simulink model "sampleModel112"  (Simulink 9.1)
settings: Solver=VariableStepAuto  StartTime=0.0  StopTime=10.0  RelTol=1e-3
undefined symbols (not defined in the file): DiscIntNeverNeededParam, Newton, Raphson
libraries: simulink x44
(part 1 of 2)
settings Model: SuppressorTable="22 serialization::archive 11 0 6 0 0 1 8 0 0 0 0 6 0 0 1 0 22 sampleModel112/cfblk81 0 6 0 0 2 8 0 0 0 0 6 41 Simulink:DataType:WarningOverFlowDetected 0 0 0 6 0  0  0 0 0 0 8 20160608 0 0 0 15 23 17 0 1 40 SimulinkFixedPoint:util:Overflowoccurred 0 0 0  0  8 20160608 0 15 23 17 0 1"  Creator=DELL  LastModifiedBy=DELL
settings DataIOCC: SaveFormat=Dataset
settings OptimizationCC: LifeSpan=auto
settings DebuggingCC: UnderspecifiedInitializationDetection=Simplified  MergeDetectMultiDrivingBlocksExec=error  SFUnexpectedBacktrackingDiag=error  SFNoUnconditionalDefaultTransitionDiag=error  SFExecutionAtInitializationDiag=warning
settings HardwareCC: ProdBitPerPointer=64  ProdBitPerSizeT=64  ProdBitPerPtrDiffT=64  ProdLargestAtomicFloat=Float  ProdIntDivRoundTo=Zero  ProdEndianess=LittleEndian  ProdWordSize=64  ProdHWDeviceType=Intel->x86-64 (Windows64)
settings ModelReferenceCC: PropagateSignalLabelsOutOfModel=on
settings CodeAppCC: StateflowObjectComments=off
settings GRTTargetCC: TargetLangStandard=C99 (ISO)  CombineOutputUpdateFcns=on  GRTInterface=off
settings ConfigComp: CovMetricSettings=dwe  CovHtmlReporting=off  CovSaveCumulativeToWorkspaceVar=off  CovSaveSingleToWorkspaceVar=off  CovExternalEMLEnable=on

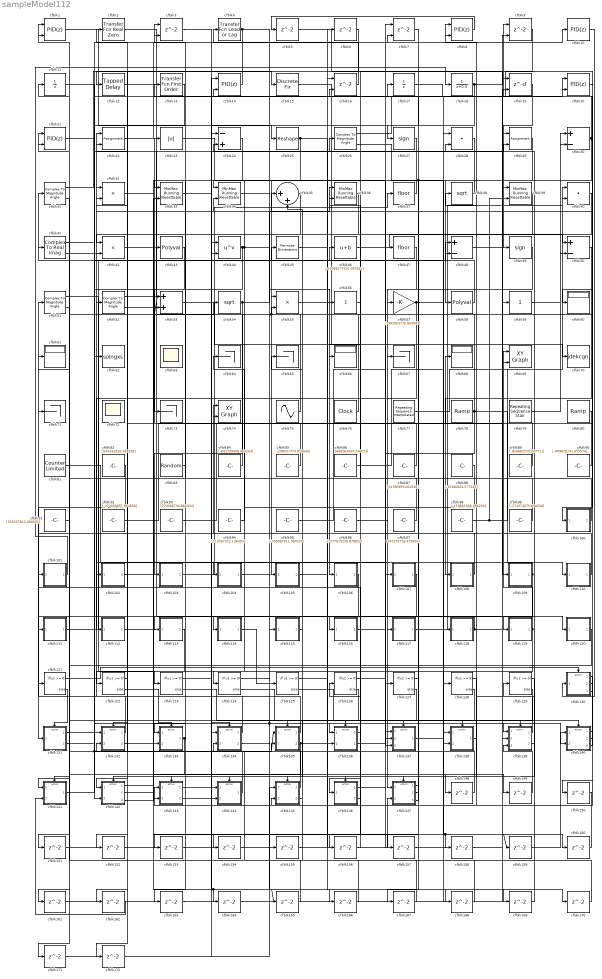
== system sampleModel112 ==
  cfblk{1,8,14,20..21} (5 alike) : simulink/Continuous/PID Controller (2DOF)  Controller=PID  TimeDomain=Discrete-time  SampleTime=1  IntegratorMethod=Forward Euler  FilterMethod=Forward Euler  Form=Parallel  UseFilter=on  ControllerParametersSource=internal  P=1  I=1  D=0  N=100  b=1  c=1  InitialConditionSource=internal  InitialConditionForIntegrator=0  InitialConditionForFilter=0  ExternalReset=none  LimitOutput=off  UpperSaturationLimit=inf  LowerSaturationLimit=-inf  LinearizeAsGain=off  AntiWindupMode=none  Kb=1  TrackingMode=off  Kt=1  PParamMin=[]  PParamMax=[]  IParamMin=[]  IParamMax=[]  DParamMin=[]  DParamMax=[]  NParamMin=[]  NParamMax=[]  bParamMin=[]  bParamMax=[]  cParamMin=[]  cParamMax=[]  KbParamMin=[]  KbParamMax=[]  KtParamMin=[]  KtParamMax=[]  POutMin=[]  POutMax=[]  IOutMin=[]  IOutMax=[]  DOutMin=[]  DOutMax=[]  NOutMin=[]  NOutMax=[]  bOutMin=[]  bOutMax=[]  cOutMin=[]  cOutMax=[]  KbOutMin=[]  KbOutMax=[]  KtOutMin=[]  KtOutMax=[]  IntegratorOutMin=[]  IntegratorOutMax=[]  FilterOutMin=[]  FilterOutMax=[]  SumOutMin=[]  SumOutMax=[]  Sum1OutMin=[]  Sum1OutMax=[]  Sum2OutMin=[]  Sum2OutMax=[]  Sum3OutMin=[]  Sum3OutMax=[]  SumI1OutMin=[]  SumI1OutMax=[]  SumI2OutMin=[]  SumI2OutMax=[]  SumI3OutMin=[]  SumI3OutMax=[]  SumDOutMin=[]  SumDOutMax=[]  SaturationOutMin=[]  SaturationOutMax=[]  IntegratorContinuousStateAttributes=''  IntegratorStateMustResolveToSignalObject=off  IntegratorRTWStateStorageClass=Auto  FilterContinuousStateAttributes=''  FilterStateMustResolveToSignalObject=off  FilterRTWStateStorageClass=Auto  DifferentiatorICPrevScaledInput=0  DifferentiatorOutMin=[]  DifferentiatorOutMax=[]  FilterDiffOutCoefMin=[]  FilterDiffOutCoefMax=[]  SumDenOutMin=[]  SumDenOutMax=[]  SumNumOutMin=[]  SumNumOutMax=[]  ReciprocalOutMin=[]  ReciprocalOutMax=[]  DivideOutMin=[]  DivideOutMax=[]  TunerSelectOption=Transfer Function Based (PID Tuner App)
  cfblk10 : simulink/Continuous/PID Controller  Controller=PID  TimeDomain=Discrete-time  SampleTime=1  IntegratorMethod=Forward Euler  FilterMethod=Forward Euler  Form=Parallel  UseFilter=on  ControllerParametersSource=internal  P=1  I=1  D=0  N=100  InitialConditionSource=internal  InitialConditionForIntegrator=0  InitialConditionForFilter=0  ExternalReset=none  LimitOutput=off  UpperSaturationLimit=inf  LowerSaturationLimit=-inf  LinearizeAsGain=off  AntiWindupMode=none  Kb=1  TrackingMode=off  Kt=1  PParamMin=[]  PParamMax=[]  IParamMin=[]  IParamMax=[]  DParamMin=[]  DParamMax=[]  NParamMin=[]  NParamMax=[]  KbParamMin=[]  KbParamMax=[]  KtParamMin=[]  KtParamMax=[]  POutMin=[]  POutMax=[]  IOutMin=[]  IOutMax=[]  DOutMin=[]  DOutMax=[]  NOutMin=[]  NOutMax=[]  KbOutMin=[]  KbOutMax=[]  KtOutMin=[]  KtOutMax=[]  IntegratorOutMin=[]  IntegratorOutMax=[]  FilterOutMin=[]  FilterOutMax=[]  SumOutMin=[]  SumOutMax=[]  SumI1OutMin=[]  SumI1OutMax=[]  SumI2OutMin=[]  SumI2OutMax=[]  SumI3OutMin=[]  SumI3OutMax=[]  SumDOutMin=[]  SumDOutMax=[]  SaturationOutMin=[]  SaturationOutMax=[]  IntegratorContinuousStateAttributes=''  IntegratorStateMustResolveToSignalObject=off  IntegratorRTWStateStorageClass=Auto  FilterContinuousStateAttributes=''  FilterStateMustResolveToSignalObject=off  FilterRTWStateStorageClass=Auto  DifferentiatorICPrevScaledInput=0  DifferentiatorOutMin=[]  DifferentiatorOutMax=[]  FilterDiffOutCoefMin=[]  FilterDiffOutCoefMax=[]  SumDenOutMin=[]  SumDenOutMax=[]  SumNumOutMin=[]  SumNumOutMax=[]  ReciprocalOutMin=[]  ReciprocalOutMax=[]  DivideOutMin=[]  DivideOutMax=[]  TunerSelectOption=Transfer Function Based (PID Tuner App)
  cfblk100 : Subsystem
  cfblk101 : Subsystem
  cfblk102 : Subsystem
  cfblk103 : Subsystem
  cfblk104 : Subsystem
  cfblk105 : Subsystem
  cfblk106 : Subsystem
  cfblk107 : Subsystem
  cfblk108 : Subsystem
  cfblk109 : Subsystem
  cfblk11 : UnitDelay
  cfblk110 : Subsystem
  cfblk111 : Subsystem
  cfblk112 : Subsystem
  cfblk113 : Subsystem
  cfblk114 : Subsystem
  cfblk115 : Subsystem
  cfblk116 : Subsystem
  cfblk117 : Subsystem
  cfblk118 : Subsystem
  cfblk119 : Subsystem
  cfblk12 : simulink/Discrete/Tapped Delay  vinit=0.0  samptime=-1  NumDelays=1  DelayOrder=Oldest  includeCurrent=off
  cfblk120 : Subsystem
  cfblk{121..129} (9 alike) : If  IfExpression=u1 >= 0  SampleTime=1
  cfblk13 : simulink/Discrete/Transfer Fcn First Order  PoleZ=0.95  ICPrevOutput=0.0  DoSatur=off
      settings: SourceProductName=Simulink
  cfblk130 : Subsystem  TreatAsAtomicUnit=on
  cfblk131 : Subsystem  TreatAsAtomicUnit=on
  cfblk132 : Subsystem  TreatAsAtomicUnit=on
  cfblk133 : Subsystem  TreatAsAtomicUnit=on
  cfblk134 : Subsystem  TreatAsAtomicUnit=on
  cfblk135 : Subsystem  TreatAsAtomicUnit=on
  cfblk136 : Subsystem  TreatAsAtomicUnit=on
  cfblk137 : Subsystem  TreatAsAtomicUnit=on
  cfblk138 : Subsystem  TreatAsAtomicUnit=on
  cfblk139 : Subsystem  TreatAsAtomicUnit=on
  cfblk140 : Subsystem  TreatAsAtomicUnit=on
  cfblk141 : Subsystem  TreatAsAtomicUnit=on
  cfblk142 : Subsystem  TreatAsAtomicUnit=on
  cfblk143 : Subsystem  TreatAsAtomicUnit=on
  cfblk144 : Subsystem  TreatAsAtomicUnit=on
  cfblk145 : Subsystem  TreatAsAtomicUnit=on
  cfblk146 : Subsystem  TreatAsAtomicUnit=on
  cfblk147 : Subsystem  TreatAsAtomicUnit=on
  cfblk{5..6,148..172} (27 alike) : Delay  SampleTime=1
  cfblk15 : DiscreteFir  SampleTime=1
  cfblk{3,7,9,16} (4 alike) : Delay  ShowEnablePort=on  SampleTime=1
      settings: InputPortMap=u0,e6
  cfblk17 : UnitDelay
  cfblk18 : DiscreteTransferFcn  SampleTime=1
  cfblk19 : Delay  DelayLengthSource=Input port  SampleTime=1
      settings: InputPortMap=u0,p1
  cfblk2 : simulink/Discrete/Transfer Fcn Real Zero  ZeroZ=0.75  ICPrevInput=0.0  DoSatur=off
      settings: SourceProductName=Simulink  SourceProductBaseCode=SL
  cfblk22 : Assignment  DiagnosticForDimensions=Warning  IndexOptions=Index vector (dialog)  Indices=1  OutputSizes=1
  cfblk23 : Abs
  cfblk24 : Sum  Inputs=-+
  cfblk25 : Reshape
  cfblk{26,31,51..52} (4 alike) : ComplexToMagnitudeAngle
  cfblk27 : Signum
  cfblk28 : DotProduct  InputSameDT=on  OutDataTypeStr=Inherit: Inherit via internal rule
  cfblk29 : Assignment  DiagnosticForDimensions=Warning  IndexOptions=Index vector (dialog)  Indices=1  OutputSizes=1
  cfblk30 : Sum  Inputs=+-
  cfblk32 : Product
  cfblk{33..34,36,39} (4 alike) : simulink/Math Operations/MinMax Running Resettable  Function=min  vinit=0.0
  cfblk35 : Sum  Inputs=|++
  cfblk37 : Rounding
  cfblk38 : Sqrt  SaturateOnIntegerOverflow=on
  cfblk4 : simulink/Discrete/Transfer Fcn Lead or Lag  PoleZ=0.95  ZeroZ=0.75  ICPrevOutput=0.0  ICPrevInput=0.0  DoSatur=off
      settings: SourceProductName=Simulink  SourceProductBaseCode=SL
  cfblk40 : DotProduct  InputSameDT=on  OutDataTypeStr=Inherit: Inherit via internal rule
  cfblk41 : ComplexToRealImag
  cfblk42 : Product  Inputs=**
  cfblk43 : Polyval  Coefs=[ +2.081618890e-019, -1.441693666e-014, +4.719686976e-010, -8.536869453e-006, +1.621573104e-001, -8.087801117e+001 ]
  cfblk44 : Math  Operator=pow  SaturateOnIntegerOverflow=on
  cfblk45 : PermuteDimensions
  cfblk46 : Bias  Bias=[989277410.097821]
  cfblk47 : Rounding
  cfblk48 : Sum  Inputs=+-
  cfblk49 : Signum
  cfblk50 : Sum  Inputs=+-
  cfblk53 : Sum
  cfblk54 : Sqrt  SaturateOnIntegerOverflow=on
  cfblk55 : Product  Inputs=**
  cfblk56 : Sum  Inputs=+
  cfblk57 : Gain  Gain=[-992003770.603943]
  cfblk58 : Polyval  Coefs=[ +2.081618890e-019, -1.441693666e-014, +4.719686976e-010, -8.536869453e-006, +1.621573104e-001, -8.087801117e+001 ]
  cfblk59 : simulink/Math Operations/Slider Gain  gain=1  low=0  high=2
  cfblk{60..61,66,68} (4 alike) : Display
  cfblk62 : ToWorkspace  VariableName=solngxs  SaveFormat=Timeseries  SampleTime=-1
  cfblk63 : Scope
      settings: Floating=on
  cfblk{64..65,67,71,73} (5 alike) : Terminator
  cfblk69 : simulink/Sinks/XY Graph  xmin=-1  xmax=1  ymin=-1  ymax=1  st=-1
  cfblk70 : ToWorkspace  VariableName=jdekcgn  SaveFormat=Timeseries  SampleTime=-1
  cfblk72 : Scope
      settings: Floating=on
  cfblk74 : simulink/Sinks/XY Graph  xmin=-1  xmax=1  ymin=-1  ymax=1  st=-1
  cfblk75 : Sin  Amplitude=[-145605885.382859]  Bias=[-797728255.211016]  SampleTime=0
  cfblk76 : DigitalClock
  cfblk77 : simulink/Sources/Repeating Sequence Interpolated  OutValues=[-370249542.565422, -774787693.113988, 675281554.388704, -493341960.193509, 181293686.473387]  TimeValues=[0 0.1 0.5 0.6 1].'  LookUpMeth=Use Input Above  tsamp=0.01  OutMin=[]  OutMax=[]  OutDataTypeStr=double  OutputDataTypeScalingMode=double  OutDataType=fixdt(0,8)  OutScaling=2^-10
  cfblk78 : simulink/Sources/Ramp  slope=[2818.028998]  start=[30.439824]  InitialOutput=[315717.012690]
  cfblk79 : simulink/Sources/Repeating Sequence Stair  OutValues=[132599061.622461, -803275858.841919]  tsamp=-1  OutMin=[]  OutMax=[]  OutDataTypeStr=double  OutputDataTypeScalingMode=double  OutDataType=fixdt(0,8)  ConRadixGroup=Best Precision: Vector-wise  OutScaling=2^-12
  cfblk80 : simulink/Sources/Ramp  slope=[-5793.235328]  start=[14.690566]  InitialOutput=[133772.427561]
  cfblk81 : simulink/Sources/Counter Limited  uplimit=[276.000000]  tsamp=-1
  cfblk82 : Constant  Value=[639181520.339358]  SampleTime=1
  cfblk83 : UniformRandomNumber  Minimum=[-8236368095.741834]  Maximum=[8276593604.768766]  Seed=[22727342.000000]  SampleTime=0.1
  cfblk84 : Constant  Value=[-641739458.403204]  SampleTime=1
  cfblk85 : Constant  Value=[298537775.810636]  SampleTime=1
  cfblk86 : Constant  Value=[448583934.246073]  SampleTime=1
  cfblk87 : Constant  Value=[54786959.062546]  SampleTime=1
  cfblk88 : Constant  Value=[-19180664.577623]  SampleTime=1
  cfblk89 : Constant  Value=[-826682570.047711]  SampleTime=1
  cfblk90 : Constant  Value=[-989820241.655576]  SampleTime=1
  cfblk91 : Constant  Value=[555557812.090935]  SampleTime=1
  cfblk92 : Constant  Value=[-274050697.954858]  SampleTime=1
  cfblk93 : Constant  Value=[270266734.884034]  SampleTime=1
  cfblk94 : Constant  Value=[113067322.136453]  SampleTime=1
  cfblk95 : Constant  Value=[-750967911.584239]  SampleTime=1
  cfblk96 : Constant  Value=[-277615226.876852]  SampleTime=1
  cfblk97 : Constant  Value=[497279716.475859]  SampleTime=1
  cfblk98 : Constant  Value=[-119851956.386200]  SampleTime=1
  cfblk99 : Constant  Value=[-174374075.858508]  SampleTime=1
  wires:
  cfblk27/1 -> cfblk105/1(cfblk1)
  cfblk12/1 -> cfblk120/1(cfblk1)
  cfblk114/1(cfblk2) -> cfblk125/1
  cfblk132/1(cfblk2) -> cfblk22/1
  cfblk77/1 -> cfblk40/1
  cfblk108/1(cfblk2) -> cfblk51/1
  cfblk31/1 -> cfblk15/1
  cfblk37/1 -> cfblk34/1
  cfblk113/1(cfblk2) -> cfblk122/1
  cfblk96/1 -> cfblk147/1(cfblk1)
  cfblk54/1 -> cfblk103/1(cfblk1), cfblk36/2
  cfblk55/1 -> cfblk106/1(cfblk1)
  cfblk47/1 -> cfblk117/1(cfblk1)
  cfblk19/1 -> cfblk49/1
  cfblk101/1(cfblk2) -> cfblk18/1
  cfblk143/1(cfblk2) -> cfblk17/1
  cfblk102/1(cfblk2) -> cfblk164/1, cfblk165/1
  cfblk16/1 -> cfblk4/1
  cfblk81/1 -> cfblk127/1
  cfblk117/1(cfblk2) -> cfblk40/2
  cfblk53/1 -> cfblk67/1
  cfblk38/1 -> cfblk58/1
  cfblk92/1 -> cfblk68/1
  cfblk140/1(cfblk2) -> cfblk143/1(cfblk1)
  cfblk30/1 -> cfblk143/2(cfblk14), cfblk16/2
  cfblk103/1(cfblk2) -> cfblk37/1
  cfblk17/1 -> cfblk100/1(cfblk1)
  cfblk1/1 -> cfblk115/1(cfblk1)
  cfblk15/1 -> cfblk70/1
  cfblk9/1 -> cfblk66/1
  cfblk35/1 -> cfblk42/1
  cfblk111/1(cfblk2) -> cfblk48/1
  cfblk26/1 -> cfblk9/1
  cfblk131/1(cfblk2) -> cfblk132/1(cfblk1)
  cfblk2/1 -> cfblk25/1
  cfblk146/1(cfblk2) -> cfblk137/1(cfblk1)
  cfblk82/1 -> cfblk131/1(cfblk1)
  cfblk134/1(cfblk2) -> cfblk71/1
  cfblk7/1 -> cfblk27/1
  cfblk105/1(cfblk2) -> cfblk48/2
  cfblk86/1 -> cfblk28/1
  cfblk97/1 -> cfblk46/1
  cfblk20/1 -> cfblk60/1
  cfblk58/1 -> cfblk31/1
  cfblk109/1(cfblk2) -> cfblk121/1, cfblk102/1(cfblk1)
  cfblk107/1(cfblk2) -> cfblk111/1(cfblk1)
  cfblk110/1(cfblk2) -> cfblk74/1
  cfblk23/1 -> cfblk107/1(cfblk1)
  cfblk89/1 -> cfblk36/1
  cfblk79/1 -> cfblk30/1
  cfblk85/1 -> cfblk23/1
  cfblk14/1 -> cfblk12/1
  cfblk4/1 -> cfblk56/1, cfblk152/1
  cfblk39/1 -> cfblk146/1(cfblk1)
  cfblk138/1(cfblk2) -> cfblk38/1
  cfblk84/1 -> cfblk32/1
  cfblk8/1 -> cfblk5/1
  cfblk51/1 -> cfblk123/1
  cfblk3/1 -> cfblk119/1(cfblk1)
  cfblk25/1 -> cfblk144/2(cfblk9), cfblk140/2(cfblk11)
  cfblk146/2(cfblk7) -> cfblk101/1(cfblk1)
  cfblk99/1 -> cfblk3/1
  cfblk51/2 -> cfblk11/1
  cfblk43/1 -> cfblk73/1
  cfblk143/2(cfblk15) -> cfblk14/1
  cfblk147/3(cfblk14) -> cfblk13/1
  cfblk10/1 -> cfblk130/1(cfblk1)
  cfblk46/1 -> cfblk50/1
  cfblk48/1 -> cfblk59/1
  cfblk40/1 -> cfblk55/1
  cfblk50/1 -> cfblk108/1(cfblk1)
  cfblk11/1 -> cfblk62/1
  cfblk13/1 -> cfblk42/2
  cfblk94/1 -> cfblk64/1
  cfblk29/1 -> cfblk104/1(cfblk1), cfblk167/1
  cfblk88/1 -> cfblk124/1
  cfblk93/1 -> cfblk69/1
  cfblk28/1 -> cfblk113/1(cfblk1)
  cfblk131/2(cfblk10) -> cfblk3/2
  cfblk119/1(cfblk2) -> cfblk69/2, cfblk133/2(cfblk7)
  cfblk87/1 -> cfblk22/2
  cfblk59/1 -> cfblk30/2
  cfblk41/1 -> cfblk136/1(cfblk1)
  cfblk115/1(cfblk2) -> cfblk35/2
  cfblk6/1 -> cfblk142/1(cfblk1)
  cfblk41/2 -> cfblk19/1
  cfblk118/1(cfblk2) -> cfblk39/1, cfblk116/1(cfblk1)
  cfblk52/1 -> cfblk26/1
  cfblk5/1 -> cfblk109/1(cfblk1)
  cfblk112/1(cfblk2) -> cfblk158/1, cfblk159/1
  cfblk136/1(cfblk2) -> cfblk132/2(cfblk14)
  cfblk44/1 -> cfblk114/1(cfblk1), cfblk139/1(cfblk1), cfblk142/2(cfblk14)
  cfblk78/1 -> cfblk110/1(cfblk1), cfblk137/3(cfblk13), cfblk53/2
  cfblk90/1 -> cfblk28/2
  cfblk76/1 -> cfblk1/1
  cfblk144/1(cfblk2) -> cfblk52/1
  cfblk98/1 -> cfblk50/2, cfblk39/2
  cfblk22/1 -> cfblk7/2
  cfblk145/1(cfblk2) -> cfblk41/1
  cfblk26/2 -> cfblk118/1(cfblk1)
  cfblk21/1 -> cfblk29/2
  cfblk116/1(cfblk2) -> cfblk10/1
  cfblk136/2(cfblk15) -> cfblk20/1
  cfblk130/2(cfblk6) -> cfblk32/2
  cfblk57/1 -> cfblk112/1(cfblk1), cfblk160/1
  cfblk95/1 -> cfblk47/1
  cfblk24/1 -> cfblk33/1
  cfblk142/1(cfblk2) -> cfblk33/2
  cfblk140/2(cfblk12) -> cfblk34/2
  cfblk75/1 -> cfblk2/1
  cfblk141/1(cfblk2) -> cfblk43/1, cfblk135/1(cfblk1)
  cfblk100/1(cfblk2) -> cfblk1/2
  cfblk145/2(cfblk15) -> cfblk65/1
  cfblk140/3(cfblk13) -> cfblk14/2
  cfblk137/1(cfblk2) -> cfblk20/2
  cfblk32/1 -> cfblk136/2(cfblk14)
  cfblk80/1 -> cfblk74/2
  cfblk142/3(cfblk16) -> cfblk45/1
  cfblk139/1(cfblk2) -> cfblk8/1
  cfblk49/1 -> cfblk57/1
  cfblk91/1 -> cfblk61/1
  cfblk52/2 -> cfblk54/1
  cfblk18/1 -> cfblk9/2, cfblk44/2
  cfblk139/2(cfblk17) -> cfblk24/2
  cfblk130/3(cfblk7) -> cfblk53/1, cfblk55/2
  cfblk135/1(cfblk2) -> cfblk21/1
  cfblk135/2(cfblk10) -> cfblk6/1, cfblk171/1
  cfblk31/2 -> cfblk141/1(cfblk1)
  cfblk104/1(cfblk2) -> cfblk137/2(cfblk12), cfblk149/1
  cfblk83/1 -> cfblk133/1(cfblk1)
  cfblk133/1(cfblk2) -> cfblk162/1, cfblk163/1
  cfblk121/1 -> cfblk130/Action
  cfblk121/2 -> cfblk131/Action
  cfblk122/1 -> cfblk132/Action
  cfblk122/2 -> cfblk133/Action
  cfblk123/1 -> cfblk134/Action
  cfblk123/2 -> cfblk135/Action
  cfblk124/1 -> cfblk136/Action
  cfblk124/2 -> cfblk137/Action
  cfblk125/1 -> cfblk138/Action
  cfblk125/2 -> cfblk139/Action
  cfblk126/1 -> cfblk140/Action
  cfblk126/2 -> cfblk141/Action
  cfblk127/1 -> cfblk142/Action
  cfblk127/2 -> cfblk143/Action
  cfblk128/1 -> cfblk144/Action
  cfblk128/2 -> cfblk145/Action
  cfblk129/1 -> cfblk146/Action
  cfblk129/2 -> cfblk147/Action
  cfblk42/1 -> cfblk148/1
  cfblk148/1 -> cfblk35/1
  cfblk149/1 -> cfblk139/3(cfblk16)
  cfblk130/1(cfblk2) -> cfblk150/1
  cfblk150/1 -> cfblk145/2(cfblk14)
  cfblk120/1(cfblk2) -> cfblk151/1
  cfblk151/1 -> cfblk128/1
  cfblk152/1 -> cfblk147/2(cfblk12)
  cfblk147/1(cfblk2) -> cfblk153/1
  cfblk153/1 -> cfblk138/2(cfblk7)
  cfblk147/2(cfblk13) -> cfblk154/1
  cfblk154/1 -> cfblk7/1
  cfblk34/1 -> cfblk155/1
  cfblk155/1 -> cfblk16/1
  cfblk56/1 -> cfblk156/1
  cfblk156/1 -> cfblk126/1
  cfblk132/2(cfblk15) -> cfblk157/1
  cfblk157/1 -> cfblk29/1
  cfblk158/1 -> cfblk19/2
  cfblk159/1 -> cfblk140/1(cfblk1)
  cfblk160/1 -> cfblk8/2
  cfblk106/1(cfblk2) -> cfblk161/1
  cfblk161/1 -> cfblk144/1(cfblk1)
  cfblk162/1 -> cfblk141/2(cfblk8)
  cfblk163/1 -> cfblk139/2(cfblk15)
  cfblk164/1 -> cfblk138/1(cfblk1)
  cfblk165/1 -> cfblk21/2
  cfblk33/1 -> cfblk166/1
  cfblk166/1 -> cfblk24/1
  cfblk167/1 -> cfblk135/2(cfblk9)
  cfblk142/2(cfblk15) -> cfblk168/1
  cfblk168/1 -> cfblk134/2(cfblk8)
  cfblk134/2(cfblk9) -> cfblk169/1
  cfblk169/1 -> cfblk129/1
  cfblk45/1 -> cfblk170/1
  cfblk170/1 -> cfblk134/1(cfblk1)
  cfblk171/1 -> cfblk44/1
  cfblk36/1 -> cfblk172/1
  cfblk172/1 -> cfblk145/1(cfblk1)

== system sampleModel112/cfblk100 ==
  cfblk1 : Inport
  cfblk2 : Outport
  wires:
  cfblk1/1 -> cfblk2/1

== system sampleModel112/cfblk101 ==
  cfblk1 : Inport
  cfblk2 : Outport
  wires:
  cfblk1/1 -> cfblk2/1

== system sampleModel112/cfblk102 ==
  cfblk1 : Inport
  cfblk2 : Outport
  wires:
  cfblk1/1 -> cfblk2/1

== system sampleModel112/cfblk103 ==
  cfblk1 : Inport
  cfblk2 : Outport
  wires:
  cfblk1/1 -> cfblk2/1

== system sampleModel112/cfblk104 ==
  cfblk1 : Inport
  cfblk2 : Outport
  wires:
  cfblk1/1 -> cfblk2/1

== system sampleModel112/cfblk105 ==
  cfblk1 : Inport
  cfblk2 : Outport
  wires:
  cfblk1/1 -> cfblk2/1

== system sampleModel112/cfblk106 ==
  cfblk1 : Inport
  cfblk2 : Outport
  wires:
  cfblk1/1 -> cfblk2/1

== system sampleModel112/cfblk107 ==
  cfblk1 : Inport
  cfblk2 : Outport
  wires:
  cfblk1/1 -> cfblk2/1

== system sampleModel112/cfblk108 ==
  cfblk1 : Inport
  cfblk2 : Outport
  wires:
  cfblk1/1 -> cfblk2/1

== system sampleModel112/cfblk109 ==
  cfblk1 : Inport
  cfblk2 : Outport
  wires:
  cfblk1/1 -> cfblk2/1

== system sampleModel112/cfblk110 ==
  cfblk1 : Inport
  cfblk2 : Outport
  wires:
  cfblk1/1 -> cfblk2/1

== system sampleModel112/cfblk111 ==
  cfblk1 : Inport
  cfblk2 : Outport
  wires:
  cfblk1/1 -> cfblk2/1

== system sampleModel112/cfblk112 ==
  cfblk1 : Inport
  cfblk2 : Outport
  wires:
  cfblk1/1 -> cfblk2/1

== system sampleModel112/cfblk113 ==
  cfblk1 : Inport
  cfblk2 : Outport
  wires:
  cfblk1/1 -> cfblk2/1

== system sampleModel112/cfblk114 ==
  cfblk1 : Inport
  cfblk2 : Outport
  wires:
  cfblk1/1 -> cfblk2/1

== system sampleModel112/cfblk115 ==
  cfblk1 : Inport
  cfblk2 : Outport
  wires:
  cfblk1/1 -> cfblk2/1

== system sampleModel112/cfblk116 ==
  cfblk1 : Inport
  cfblk2 : Outport
  wires:
  cfblk1/1 -> cfblk2/1

== system sampleModel112/cfblk117 ==
  cfblk1 : Inport
  cfblk2 : Outport
  wires:
  cfblk1/1 -> cfblk2/1

== system sampleModel112/cfblk118 ==
  cfblk1 : Inport
  cfblk2 : Outport
  wires:
  cfblk1/1 -> cfblk2/1

== system sampleModel112/cfblk119 ==
  cfblk1 : Inport
  cfblk2 : Outport
  wires:
  cfblk1/1 -> cfblk2/1

== system sampleModel112/cfblk120 ==
  cfblk1 : Inport
  cfblk2 : Outport
  wires:
  cfblk1/1 -> cfblk2/1

== system sampleModel112/cfblk130 ==
  cfblk1 : Inport
  Action Port : ActionPort  ActionType=then
  cfblk3 : ComplexToRealImag
  cfblk4 : Sqrt  Operator=rSqrt  AlgorithmType=Newton-Raphson  SaturateOnIntegerOverflow=on
  cfblk5 : Subsystem
  cfblk2 : Outport
  cfblk6 : Outport  Port=2
  cfblk7 : Outport  Port=3
  wires:
  cfblk3/1 -> cfblk6/1
  cfblk5/1(cfblk2) -> cfblk7/1, cfblk4/1
  cfblk1/1 -> cfblk3/1
  cfblk4/1 -> cfblk2/1
  cfblk3/2 -> cfblk5/1(cfblk1)

== system sampleModel112/cfblk131 ==
  cfblk1 : Inport
  Action Port : ActionPort  ActionType=else
  cfblk11 : Subsystem  TreatAsAtomicUnit=on
  cfblk12 : Subsystem  TreatAsAtomicUnit=on
  cfblk13 : Delay
  cfblk14 : Delay
  cfblk3 : DiscreteTransferFcn
  cfblk4 : simulink/Discrete/Transfer Fcn First Order  PoleZ=0.95  ICPrevOutput=0.0  DoSatur=off
      settings: SourceProductName=Simulink
  cfblk5 : ComplexToMagnitudeAngle
  cfblk6 : Constant  Value=[612674043.755625]  SampleTime=1
  cfblk7 : Subsystem
  cfblk8 : Subsystem
  cfblk9 : If  IfExpression=u1 >= 0  SampleTime=1
  cfblk2 : Outport
  cfblk10 : Outport  Port=2
  wires:
  cfblk4/1 -> cfblk7/1(cfblk1)
  cfblk7/1(cfblk2) -> cfblk3/1
  cfblk1/1 -> cfblk10/1
  cfblk5/1 -> cfblk4/1
  cfblk6/1 -> cfblk2/1, cfblk5/1
  cfblk11/1(cfblk2) -> cfblk8/1(cfblk1)
  cfblk3/1 -> cfblk12/1(cfblk1)
  cfblk5/2 -> cfblk12/2(cfblk8)
  cfblk9/1 -> cfblk11/Action
  cfblk9/2 -> cfblk12/Action
  cfblk8/1(cfblk2) -> cfblk13/1
  cfblk13/1 -> cfblk11/1(cfblk1)
  cfblk12/1(cfblk2) -> cfblk14/1
  cfblk14/1 -> cfblk9/1

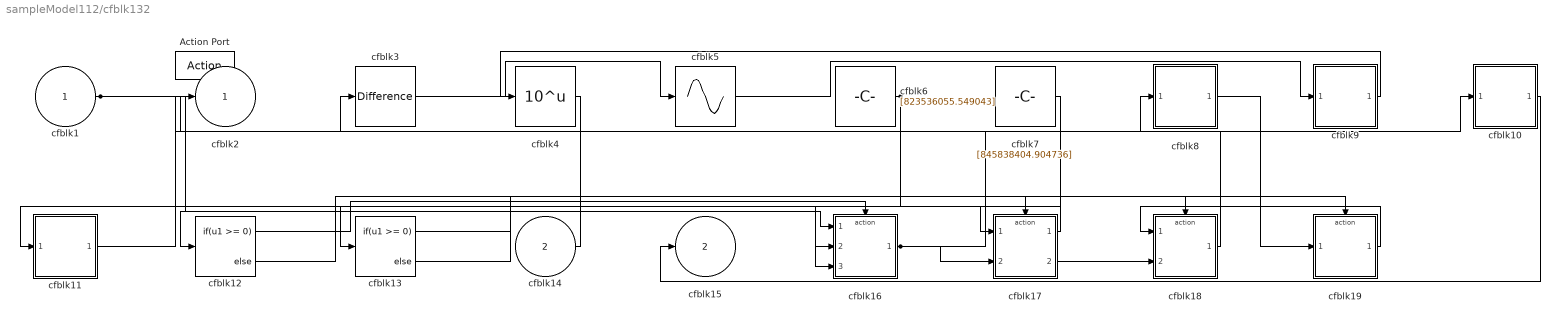
== system sampleModel112/cfblk132 ==
  cfblk1 : Inport
  cfblk14 : Inport  Port=2
  Action Port : ActionPort  ActionType=then
  cfblk10 : Subsystem
  cfblk11 : Subsystem
  cfblk12 : If  IfExpression=u1 >= 0  SampleTime=1
  cfblk13 : If  IfExpression=u1 >= 0  SampleTime=1
  cfblk16 : Subsystem  TreatAsAtomicUnit=on
  cfblk17 : Subsystem  TreatAsAtomicUnit=on
  cfblk18 : Subsystem  TreatAsAtomicUnit=on
  cfblk19 : Subsystem  TreatAsAtomicUnit=on
  cfblk3 : simulink/Discrete/Difference  ICPrevInput=0.0  OutMin=[]  OutMax=[]  OutDataTypeStr=Inherit: Inherit via back propagation  OutDataType=fixdt(1, 16)  OutScaling=2^-10  DoSatur=off
  cfblk4 : Math  Operator=10^u  SaturateOnIntegerOverflow=on
  cfblk5 : Sin  TimeSource=Use external signal  SampleTime=0
  cfblk6 : Constant  Value=[823536055.549043]  SampleTime=1
  cfblk7 : Constant  Value=[845838404.904736]  SampleTime=1
  cfblk8 : Subsystem
  cfblk9 : Subsystem
  cfblk2 : Outport
  cfblk15 : Outport  Port=2
  wires:
  cfblk1/1 -> cfblk16/1(cfblk1), cfblk17/1(cfblk1)
  cfblk10/1(cfblk2) -> cfblk15/1
  cfblk5/1 -> cfblk9/1(cfblk1)
  cfblk8/1(cfblk2) -> cfblk19/1(cfblk1)
  cfblk3/1 -> cfblk5/1
  cfblk4/1 -> cfblk12/1
  cfblk18/1(cfblk2) -> cfblk2/1
  cfblk9/1(cfblk2) -> cfblk4/1
  cfblk6/1 -> cfblk11/1(cfblk1), cfblk16/3(cfblk16)
  cfblk11/1(cfblk2) -> cfblk8/1(cfblk1)
  cfblk19/1(cfblk2) -> cfblk18/1(cfblk1)
  cfblk17/1(cfblk2) -> cfblk13/1
  cfblk14/1 -> cfblk3/1
  cfblk17/2(cfblk9) -> cfblk18/2(cfblk9)
  cfblk16/1(cfblk2) -> cfblk10/1(cfblk1), cfblk17/2(cfblk8)
  cfblk7/1 -> cfblk16/2(cfblk15)
  cfblk12/1 -> cfblk16/Action
  cfblk12/2 -> cfblk17/Action
  cfblk13/1 -> cfblk18/Action
  cfblk13/2 -> cfblk19/Action

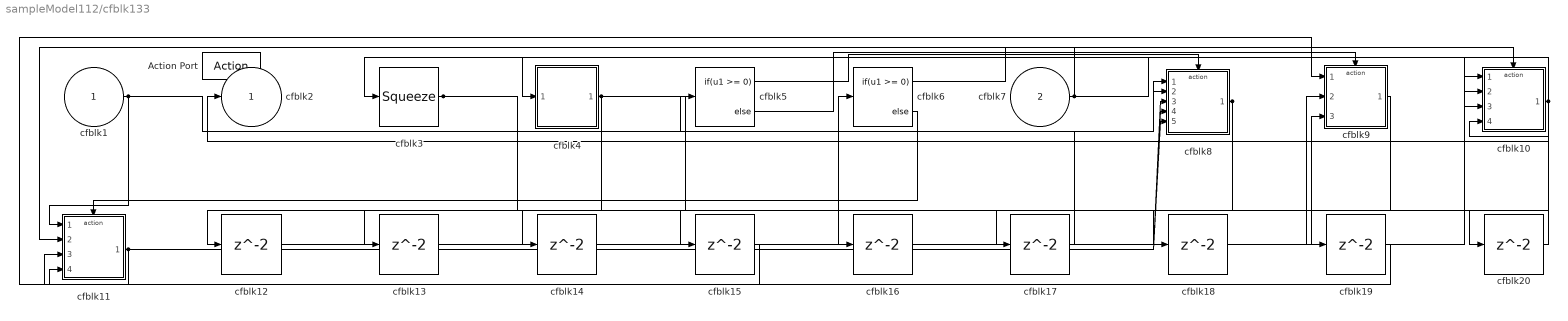
== system sampleModel112/cfblk133 ==
  cfblk1 : Inport
  cfblk7 : Inport  Port=2
  Action Port : ActionPort  ActionType=else
  cfblk10 : Subsystem  TreatAsAtomicUnit=on
  cfblk11 : Subsystem  TreatAsAtomicUnit=on
  cfblk{12..20} (9 alike) : Delay
  cfblk3 : Squeeze
  cfblk4 : Subsystem
  cfblk5 : If  IfExpression=u1 >= 0  SampleTime=1
  cfblk6 : If  IfExpression=u1 >= 0  SampleTime=1
  cfblk8 : Subsystem  TreatAsAtomicUnit=on
  cfblk9 : Subsystem  TreatAsAtomicUnit=on
  cfblk2 : Outport
  wires:
  cfblk1/1 -> cfblk11/1(cfblk1), cfblk8/1(cfblk1), cfblk8/2(cfblk12)
  cfblk10/1(cfblk2) -> cfblk2/1, cfblk4/1(cfblk1), cfblk3/1, cfblk13/1
  cfblk4/1(cfblk2) -> cfblk14/1, cfblk17/1
  cfblk7/1 -> cfblk11/2(cfblk8), cfblk10/2(cfblk8)
  cfblk8/1(cfblk2) -> cfblk15/1, cfblk16/1
  cfblk11/1(cfblk2) -> cfblk9/1(cfblk1), cfblk8/3(cfblk13), cfblk8/4(cfblk14), cfblk8/5(cfblk15)
  cfblk3/1 -> cfblk18/1, cfblk19/1, cfblk20/1
  cfblk5/1 -> cfblk8/Action
  cfblk5/2 -> cfblk9/Action
  cfblk6/1 -> cfblk10/Action
  cfblk6/2 -> cfblk11/Action
  cfblk9/1(cfblk2) -> cfblk12/1
  cfblk12/1 -> cfblk10/1(cfblk1)
  cfblk13/1 -> cfblk9/3(cfblk7)
  cfblk14/1 -> cfblk6/1
  cfblk15/1 -> cfblk11/3(cfblk9)
  cfblk16/1 -> cfblk10/3(cfblk9)
  cfblk17/1 -> cfblk5/1
  cfblk18/1 -> cfblk9/2(cfblk6)
  cfblk19/1 -> cfblk11/4(cfblk10)
  cfblk20/1 -> cfblk10/4(cfblk10)

== system sampleModel112/cfblk134 ==
  cfblk1 : Inport
  cfblk8 : Inport  Port=2
  Action Port : ActionPort  ActionType=then
  cfblk3 : simulink/Discrete/Tapped Delay  vinit=0.0  samptime=-1  NumDelays=1  DelayOrder=Oldest  includeCurrent=off
  cfblk4 : simulink/Continuous/PID Controller (2DOF)  Controller=PID  TimeDomain=Discrete-time  SampleTime=-1  IntegratorMethod=Forward Euler  FilterMethod=Forward Euler  Form=Parallel  UseFilter=on  ControllerParametersSource=internal  P=1  I=1  D=0  N=100  b=1  c=1  InitialConditionSource=internal  InitialConditionForIntegrator=0  InitialConditionForFilter=0  ExternalReset=none  LimitOutput=off  UpperSaturationLimit=inf  LowerSaturationLimit=-inf  LinearizeAsGain=off  AntiWindupMode=none  Kb=1  TrackingMode=off  Kt=1  PParamMin=[]  PParamMax=[]  IParamMin=[]  IParamMax=[]  DParamMin=[]  DParamMax=[]  NParamMin=[]  NParamMax=[]  bParamMin=[]  bParamMax=[]  cParamMin=[]  cParamMax=[]  KbParamMin=[]  KbParamMax=[]  KtParamMin=[]  KtParamMax=[]  POutMin=[]  POutMax=[]  IOutMin=[]  IOutMax=[]  DOutMin=[]  DOutMax=[]  NOutMin=[]  NOutMax=[]  bOutMin=[]  bOutMax=[]  cOutMin=[]  cOutMax=[]  KbOutMin=[]  KbOutMax=[]  KtOutMin=[]  KtOutMax=[]  IntegratorOutMin=[]  IntegratorOutMax=[]  FilterOutMin=[]  FilterOutMax=[]  SumOutMin=[]  SumOutMax=[]  Sum1OutMin=[]  Sum1OutMax=[]  Sum2OutMin=[]  Sum2OutMax=[]  Sum3OutMin=[]  Sum3OutMax=[]  SumI1OutMin=[]  SumI1OutMax=[]  SumI2OutMin=[]  SumI2OutMax=[]  SumI3OutMin=[]  SumI3OutMax=[]  SumDOutMin=[]  SumDOutMax=[]  SaturationOutMin=[]  SaturationOutMax=[]  IntegratorContinuousStateAttributes=''  IntegratorStateMustResolveToSignalObject=off  IntegratorRTWStateStorageClass=Auto  FilterContinuousStateAttributes=''  FilterStateMustResolveToSignalObject=off  FilterRTWStateStorageClass=Auto  DifferentiatorICPrevScaledInput=0  DifferentiatorOutMin=[]  DifferentiatorOutMax=[]  FilterDiffOutCoefMin=[]  FilterDiffOutCoefMax=[]  SumDenOutMin=[]  SumDenOutMax=[]  SumNumOutMin=[]  SumNumOutMax=[]  ReciprocalOutMin=[]  ReciprocalOutMax=[]  DivideOutMin=[]  DivideOutMax=[]  TunerSelectOption=Transfer Function Based (PID Tuner App)
  cfblk5 : Rounding
  cfblk6 : Subsystem
  cfblk7 : Subsystem
  cfblk2 : Outport
  cfblk9 : Outport  Port=2
  wires:
  cfblk8/1 -> cfblk4/1, cfblk6/1(cfblk1)
  cfblk1/1 -> cfblk7/1(cfblk1)
  cfblk6/1(cfblk2) -> cfblk4/2
  cfblk5/1 -> cfblk2/1
  cfblk4/1 -> cfblk5/1
  cfblk7/1(cfblk2) -> cfblk3/1
  cfblk3/1 -> cfblk9/1

== system sampleModel112/cfblk135 ==
  cfblk1 : Inport
  cfblk9 : Inport  Port=2
  Action Port : ActionPort  ActionType=else
  cfblk3 : simulink/Discrete/Transfer Fcn First Order  PoleZ=0.95  ICPrevOutput=0.0  DoSatur=off
      settings: SourceProductName=Simulink
  cfblk4 : simulink/Continuous/PID Controller  Controller=PID  TimeDomain=Discrete-time  SampleTime=-1  IntegratorMethod=Forward Euler  FilterMethod=Forward Euler  Form=Parallel  UseFilter=on  ControllerParametersSource=internal  P=1  I=1  D=0  N=100  InitialConditionSource=internal  InitialConditionForIntegrator=0  InitialConditionForFilter=0  ExternalReset=none  LimitOutput=off  UpperSaturationLimit=inf  LowerSaturationLimit=-inf  LinearizeAsGain=off  AntiWindupMode=none  Kb=1  TrackingMode=off  Kt=1  PParamMin=[]  PParamMax=[]  IParamMin=[]  IParamMax=[]  DParamMin=[]  DParamMax=[]  NParamMin=[]  NParamMax=[]  KbParamMin=[]  KbParamMax=[]  KtParamMin=[]  KtParamMax=[]  POutMin=[]  POutMax=[]  IOutMin=[]  IOutMax=[]  DOutMin=[]  DOutMax=[]  NOutMin=[]  NOutMax=[]  KbOutMin=[]  KbOutMax=[]  KtOutMin=[]  KtOutMax=[]  IntegratorOutMin=[]  IntegratorOutMax=[]  FilterOutMin=[]  FilterOutMax=[]  SumOutMin=[]  SumOutMax=[]  SumI1OutMin=[]  SumI1OutMax=[]  SumI2OutMin=[]  SumI2OutMax=[]  SumI3OutMin=[]  SumI3OutMax=[]  SumDOutMin=[]  SumDOutMax=[]  SaturationOutMin=[]  SaturationOutMax=[]  IntegratorContinuousStateAttributes=''  IntegratorStateMustResolveToSignalObject=off  IntegratorRTWStateStorageClass=Auto  FilterContinuousStateAttributes=''  FilterStateMustResolveToSignalObject=off  FilterRTWStateStorageClass=Auto  DifferentiatorICPrevScaledInput=0  DifferentiatorOutMin=[]  DifferentiatorOutMax=[]  FilterDiffOutCoefMin=[]  FilterDiffOutCoefMax=[]  SumDenOutMin=[]  SumDenOutMax=[]  SumNumOutMin=[]  SumNumOutMax=[]  ReciprocalOutMin=[]  ReciprocalOutMax=[]  DivideOutMin=[]  DivideOutMax=[]  TunerSelectOption=Transfer Function Based (PID Tuner App)
  cfblk5 : Sum  Inputs=|++
  cfblk6 : Constant  Value=[590020841.154756]  SampleTime=1
  cfblk7 : Subsystem
  cfblk8 : Subsystem
  cfblk2 : Outport
  cfblk10 : Outport  Port=2
  wires:
  cfblk3/1 -> cfblk7/1(cfblk1), cfblk5/2
  cfblk1/1 -> cfblk10/1
  cfblk4/1 -> cfblk8/1(cfblk1)
  cfblk9/1 -> cfblk3/1
  cfblk6/1 -> cfblk4/1
  cfblk7/1(cfblk2) -> cfblk2/1
  cfblk8/1(cfblk2) -> cfblk5/1

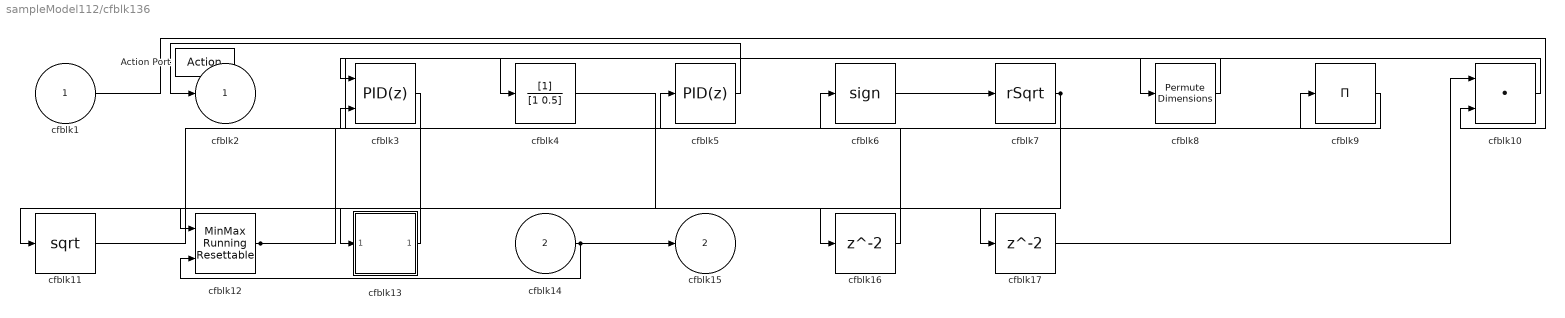
== system sampleModel112/cfblk136 ==
  cfblk1 : Inport
  cfblk14 : Inport  Port=2
  Action Port : ActionPort  ActionType=then
  cfblk10 : DotProduct  InputSameDT=on  OutDataTypeStr=Inherit: Inherit via internal rule
  cfblk11 : Sqrt  SaturateOnIntegerOverflow=on
  cfblk12 : simulink/Math Operations/MinMax Running Resettable  Function=min  vinit=0.0
  cfblk13 : Subsystem
  cfblk16 : Delay
  cfblk17 : Delay
  cfblk3 : simulink/Continuous/PID Controller (2DOF)  Controller=PID  TimeDomain=Discrete-time  SampleTime=-1  IntegratorMethod=Forward Euler  FilterMethod=Forward Euler  Form=Parallel  UseFilter=on  ControllerParametersSource=internal  P=1  I=1  D=0  N=100  b=1  c=1  InitialConditionSource=internal  InitialConditionForIntegrator=0  InitialConditionForFilter=0  ExternalReset=none  LimitOutput=off  UpperSaturationLimit=inf  LowerSaturationLimit=-inf  LinearizeAsGain=off  AntiWindupMode=none  Kb=1  TrackingMode=off  Kt=1  PParamMin=[]  PParamMax=[]  IParamMin=[]  IParamMax=[]  DParamMin=[]  DParamMax=[]  NParamMin=[]  NParamMax=[]  bParamMin=[]  bParamMax=[]  cParamMin=[]  cParamMax=[]  KbParamMin=[]  KbParamMax=[]  KtParamMin=[]  KtParamMax=[]  POutMin=[]  POutMax=[]  IOutMin=[]  IOutMax=[]  DOutMin=[]  DOutMax=[]  NOutMin=[]  NOutMax=[]  bOutMin=[]  bOutMax=[]  cOutMin=[]  cOutMax=[]  KbOutMin=[]  KbOutMax=[]  KtOutMin=[]  KtOutMax=[]  IntegratorOutMin=[]  IntegratorOutMax=[]  FilterOutMin=[]  FilterOutMax=[]  SumOutMin=[]  SumOutMax=[]  Sum1OutMin=[]  Sum1OutMax=[]  Sum2OutMin=[]  Sum2OutMax=[]  Sum3OutMin=[]  Sum3OutMax=[]  SumI1OutMin=[]  SumI1OutMax=[]  SumI2OutMin=[]  SumI2OutMax=[]  SumI3OutMin=[]  SumI3OutMax=[]  SumDOutMin=[]  SumDOutMax=[]  SaturationOutMin=[]  SaturationOutMax=[]  IntegratorContinuousStateAttributes=''  IntegratorStateMustResolveToSignalObject=off  IntegratorRTWStateStorageClass=Auto  FilterContinuousStateAttributes=''  FilterStateMustResolveToSignalObject=off  FilterRTWStateStorageClass=Auto  DifferentiatorICPrevScaledInput=0  DifferentiatorOutMin=[]  DifferentiatorOutMax=[]  FilterDiffOutCoefMin=[]  FilterDiffOutCoefMax=[]  SumDenOutMin=[]  SumDenOutMax=[]  SumNumOutMin=[]  SumNumOutMax=[]  ReciprocalOutMin=[]  ReciprocalOutMax=[]  DivideOutMin=[]  DivideOutMax=[]  TunerSelectOption=Transfer Function Based (PID Tuner App)
  cfblk4 : DiscreteFilter
  cfblk5 : simulink/Continuous/PID Controller  Controller=PID  TimeDomain=Discrete-time  SampleTime=-1  IntegratorMethod=Forward Euler  FilterMethod=Forward Euler  Form=Parallel  UseFilter=on  ControllerParametersSource=internal  P=1  I=1  D=0  N=100  InitialConditionSource=internal  InitialConditionForIntegrator=0  InitialConditionForFilter=0  ExternalReset=none  LimitOutput=off  UpperSaturationLimit=inf  LowerSaturationLimit=-inf  LinearizeAsGain=off  AntiWindupMode=none  Kb=1  TrackingMode=off  Kt=1  PParamMin=[]  PParamMax=[]  IParamMin=[]  IParamMax=[]  DParamMin=[]  DParamMax=[]  NParamMin=[]  NParamMax=[]  KbParamMin=[]  KbParamMax=[]  KtParamMin=[]  KtParamMax=[]  POutMin=[]  POutMax=[]  IOutMin=[]  IOutMax=[]  DOutMin=[]  DOutMax=[]  NOutMin=[]  NOutMax=[]  KbOutMin=[]  KbOutMax=[]  KtOutMin=[]  KtOutMax=[]  IntegratorOutMin=[]  IntegratorOutMax=[]  FilterOutMin=[]  FilterOutMax=[]  SumOutMin=[]  SumOutMax=[]  SumI1OutMin=[]  SumI1OutMax=[]  SumI2OutMin=[]  SumI2OutMax=[]  SumI3OutMin=[]  SumI3OutMax=[]  SumDOutMin=[]  SumDOutMax=[]  SaturationOutMin=[]  SaturationOutMax=[]  IntegratorContinuousStateAttributes=''  IntegratorStateMustResolveToSignalObject=off  IntegratorRTWStateStorageClass=Auto  FilterContinuousStateAttributes=''  FilterStateMustResolveToSignalObject=off  FilterRTWStateStorageClass=Auto  DifferentiatorICPrevScaledInput=0  DifferentiatorOutMin=[]  DifferentiatorOutMax=[]  FilterDiffOutCoefMin=[]  FilterDiffOutCoefMax=[]  SumDenOutMin=[]  SumDenOutMax=[]  SumNumOutMin=[]  SumNumOutMax=[]  ReciprocalOutMin=[]  ReciprocalOutMax=[]  DivideOutMin=[]  DivideOutMax=[]  TunerSelectOption=Transfer Function Based (PID Tuner App)
  cfblk6 : Signum
  cfblk7 : Sqrt  Operator=rSqrt  AlgorithmType=Newton-Raphson  SaturateOnIntegerOverflow=on
  cfblk8 : PermuteDimensions
  cfblk9 : Product  Inputs=*
  cfblk2 : Outport
  cfblk15 : Outport  Port=2
  wires:
  cfblk14/1 -> cfblk15/1, cfblk12/2
  cfblk6/1 -> cfblk7/1
  cfblk3/1 -> cfblk13/1(cfblk1)
  cfblk11/1 -> cfblk4/1
  cfblk13/1(cfblk2) -> cfblk12/1
  cfblk5/1 -> cfblk2/1
  cfblk10/1 -> cfblk8/1
  cfblk9/1 -> cfblk5/1
  cfblk12/1 -> cfblk6/1, cfblk9/1
  cfblk8/1 -> cfblk3/1
  cfblk7/1 -> cfblk11/1, cfblk16/1
  cfblk1/1 -> cfblk10/2
  cfblk16/1 -> cfblk3/2
  cfblk4/1 -> cfblk17/1
  cfblk17/1 -> cfblk10/1

== system sampleModel112/cfblk137 ==
  cfblk1 : Inport
  cfblk12 : Inport  Port=2
  cfblk13 : Inport  Port=3
  Action Port : ActionPort  ActionType=else
  cfblk10 : Subsystem
  cfblk11 : Subsystem
  cfblk3 : Reshape
  cfblk4 : Reshape
  cfblk5 : Squeeze
  cfblk6 : Sqrt  SaturateOnIntegerOverflow=on
  cfblk7 : UnaryMinus
  cfblk8 : DotProduct  InputSameDT=on  OutDataTypeStr=Inherit: Inherit via internal rule
  cfblk9 : Constant  Value=[-603563242.963651]  SampleTime=1
  cfblk2 : Outport
  wires:
  cfblk13/1 -> cfblk7/1
  cfblk1/1 -> cfblk10/1(cfblk1)
  cfblk11/1(cfblk2) -> cfblk4/1
  cfblk5/1 -> cfblk2/1
  cfblk7/1 -> cfblk8/1
  cfblk6/1 -> cfblk3/1
  cfblk3/1 -> cfblk5/1
  cfblk4/1 -> cfblk8/2
  cfblk10/1(cfblk2) -> cfblk11/1(cfblk1)
  cfblk9/1 -> cfblk6/1

== system sampleModel112/cfblk138 ==
  cfblk1 : Inport
  cfblk7 : Inport  Port=2
  Action Port : ActionPort  ActionType=then
  cfblk3 : simulink/Discrete/Transfer Fcn Real Zero  ZeroZ=0.75  ICPrevInput=0.0  DoSatur=off
      settings: SourceProductName=Simulink  SourceProductBaseCode=SL
  cfblk4 : Gain  Gain=[-633442323.926628]
  cfblk5 : UnaryMinus
  cfblk6 : Subsystem
  cfblk8 : Delay
  cfblk2 : Outport
  wires:
  cfblk4/1 -> cfblk5/1
  cfblk1/1 -> cfblk3/1
  cfblk7/1 -> cfblk6/1(cfblk1)
  cfblk3/1 -> cfblk2/1
  cfblk5/1 -> cfblk8/1
  cfblk8/1 -> cfblk4/1

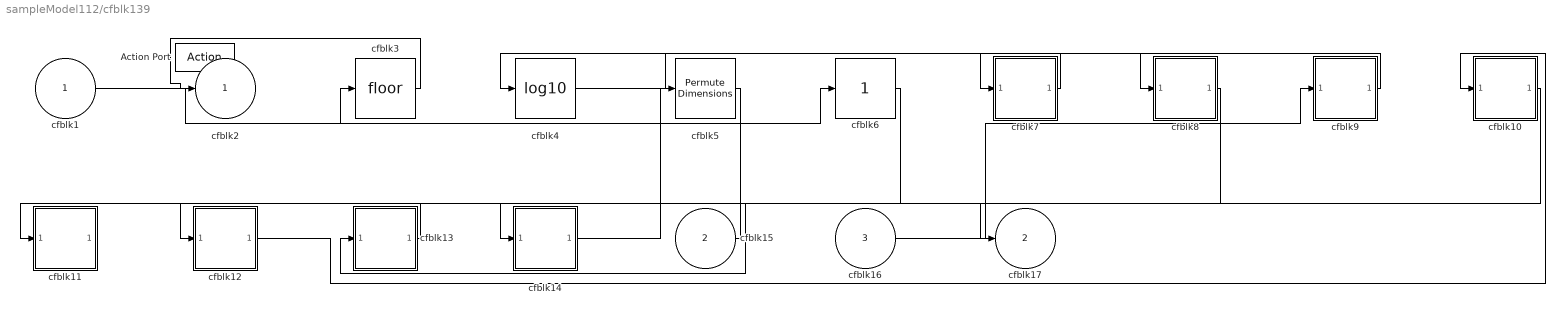
== system sampleModel112/cfblk139 ==
  cfblk1 : Inport
  cfblk15 : Inport  Port=2
  cfblk16 : Inport  Port=3
  Action Port : ActionPort  ActionType=else
  cfblk10 : Subsystem
  cfblk11 : Subsystem
  cfblk12 : Subsystem
  cfblk13 : Subsystem
  cfblk14 : Subsystem
  cfblk3 : Rounding
  cfblk4 : Math  Operator=log10  SaturateOnIntegerOverflow=on
  cfblk5 : PermuteDimensions
  cfblk6 : simulink/Math Operations/Slider Gain  gain=1  low=0  high=2
  cfblk7 : Subsystem
  cfblk8 : Subsystem
  cfblk9 : Subsystem
  cfblk2 : Outport
  cfblk17 : Outport  Port=2
  wires:
  cfblk16/1 -> cfblk9/1(cfblk1)
  cfblk15/1 -> cfblk3/1
  cfblk4/1 -> cfblk8/1(cfblk1)
  cfblk8/1(cfblk2) -> cfblk17/1
  cfblk6/1 -> cfblk13/1(cfblk1)
  cfblk13/1(cfblk2) -> cfblk12/1(cfblk1)
  cfblk14/1(cfblk2) -> cfblk5/1
  cfblk1/1 -> cfblk6/1
  cfblk10/1(cfblk2) -> cfblk14/1(cfblk1)
  cfblk5/1 -> cfblk11/1(cfblk1)
  cfblk7/1(cfblk2) -> cfblk4/1
  cfblk9/1(cfblk2) -> cfblk7/1(cfblk1)
  cfblk3/1 -> cfblk2/1
  cfblk12/1(cfblk2) -> cfblk10/1(cfblk1)

== system sampleModel112/cfblk140 ==
  cfblk1 : Inport
  cfblk11 : Inport  Port=2
  Action Port : ActionPort  ActionType=then
  cfblk10 : Subsystem
  cfblk3 : Sum  Inputs=|++
  cfblk4 : Squeeze
  cfblk5 : Constant  Value=[828235013.222920]  SampleTime=1
  cfblk6 : Constant  Value=[868174128.161214]  SampleTime=1
  cfblk7 : Subsystem
  cfblk8 : Subsystem
  cfblk9 : Subsystem
  cfblk2 : Outport
  cfblk12 : Outport  Port=2
  cfblk13 : Outport  Port=3
  wires:
  cfblk7/1(cfblk2) -> cfblk10/1(cfblk1)
  cfblk1/1 -> cfblk3/1
  cfblk5/1 -> cfblk8/1(cfblk1)
  cfblk10/1(cfblk2) -> cfblk3/2
  cfblk11/1 -> cfblk4/1
  cfblk4/1 -> cfblk9/1(cfblk1)
  cfblk8/1(cfblk2) -> cfblk7/1(cfblk1)
  cfblk6/1 -> cfblk12/1
  cfblk3/1 -> cfblk2/1
  cfblk9/1(cfblk2) -> cfblk13/1

== system sampleModel112/cfblk141 ==
  cfblk1 : Inport
  cfblk8 : Inport  Port=2
  Action Port : ActionPort  ActionType=else
  cfblk3 : Sum  Inputs=+
  cfblk4 : Constant  Value=[-338856808.742728]  SampleTime=1
  cfblk5 : Subsystem
  cfblk6 : Subsystem
  cfblk7 : Subsystem
  cfblk2 : Outport
  wires:
  cfblk4/1 -> cfblk5/1(cfblk1)
  cfblk5/1(cfblk2) -> cfblk3/1
  cfblk6/1(cfblk2) -> cfblk2/1
  cfblk3/1 -> cfblk6/1(cfblk1)
  cfblk1/1 -> cfblk7/1(cfblk1)

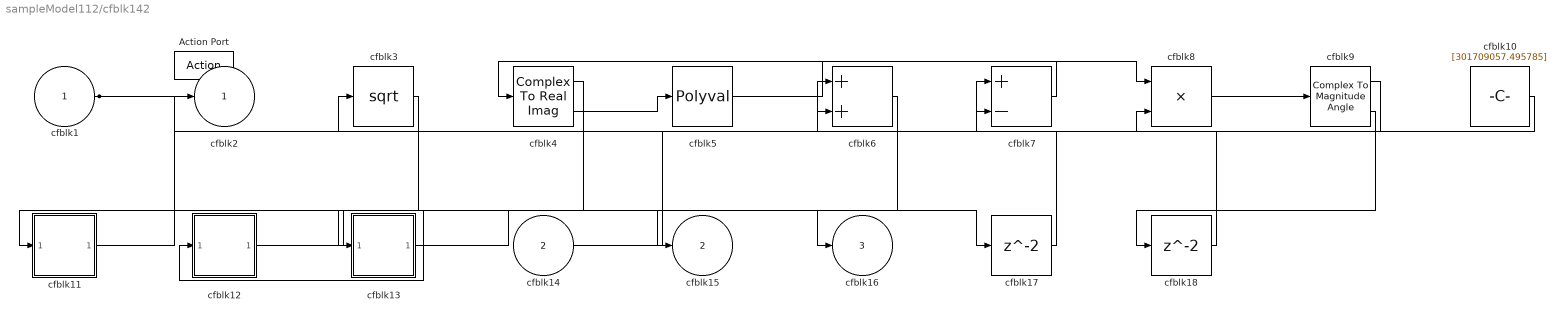
== system sampleModel112/cfblk142 ==
  cfblk1 : Inport
  cfblk14 : Inport  Port=2
  Action Port : ActionPort  ActionType=then
  cfblk10 : Constant  Value=[301709057.495785]  SampleTime=1
  cfblk11 : Subsystem
  cfblk12 : Subsystem
  cfblk13 : Subsystem
  cfblk17 : Delay
  cfblk18 : Delay
  cfblk3 : Sqrt  SaturateOnIntegerOverflow=on
  cfblk4 : ComplexToRealImag
  cfblk5 : Polyval  Coefs=[ +2.081618890e-019, -1.441693666e-014, +4.719686976e-010, -8.536869453e-006, +1.621573104e-001, -8.087801117e+001 ]
  cfblk6 : Sum
  cfblk7 : Sum  Inputs=+-
  cfblk8 : Product
  cfblk9 : ComplexToMagnitudeAngle
  cfblk2 : Outport
  cfblk15 : Outport  Port=2
  cfblk16 : Outport  Port=3
  wires:
  cfblk1/1 -> cfblk2/1, cfblk15/1
  cfblk14/1 -> cfblk7/1
  cfblk3/1 -> cfblk11/1(cfblk1)
  cfblk4/1 -> cfblk12/1(cfblk1)
  cfblk4/2 -> cfblk5/1
  cfblk7/1 -> cfblk4/1
  cfblk5/1 -> cfblk8/1
  cfblk10/1 -> cfblk7/2
  cfblk11/1(cfblk2) -> cfblk6/1
  cfblk12/1(cfblk2) -> cfblk16/1
  cfblk9/1 -> cfblk6/2
  cfblk6/1 -> cfblk13/1(cfblk1)
  cfblk8/1 -> cfblk9/1
  cfblk13/1(cfblk2) -> cfblk17/1
  cfblk17/1 -> cfblk3/1
  cfblk9/2 -> cfblk18/1
  cfblk18/1 -> cfblk8/2

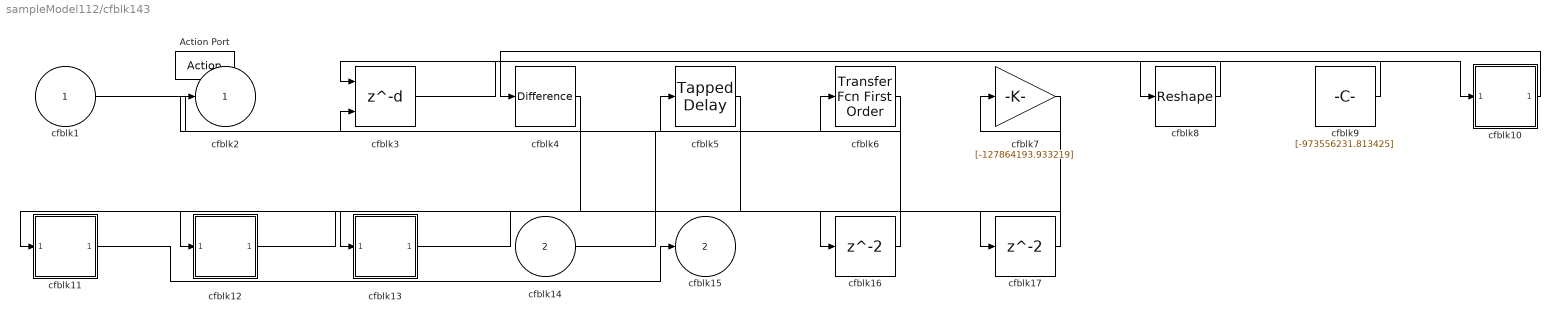
== system sampleModel112/cfblk143 ==
  cfblk1 : Inport
  cfblk14 : Inport  Port=2
  Action Port : ActionPort  ActionType=else
  cfblk10 : Subsystem
  cfblk11 : Subsystem
  cfblk12 : Subsystem
  cfblk13 : Subsystem
  cfblk16 : Delay
  cfblk17 : Delay
  cfblk3 : Delay  DelayLengthSource=Input port
      settings: InputPortMap=u0,p1
  cfblk4 : simulink/Discrete/Difference  ICPrevInput=0.0  OutMin=[]  OutMax=[]  OutDataTypeStr=Inherit: Inherit via back propagation  OutDataType=fixdt(1, 16)  OutScaling=2^-10  DoSatur=off
  cfblk5 : simulink/Discrete/Tapped Delay  vinit=0.0  samptime=-1  NumDelays=1  DelayOrder=Oldest  includeCurrent=off
  cfblk6 : simulink/Discrete/Transfer Fcn First Order  PoleZ=0.95  ICPrevOutput=0.0  DoSatur=off
      settings: SourceProductName=Simulink
  cfblk7 : Gain  Gain=[-127864193.933219]
  cfblk8 : Reshape
  cfblk9 : Constant  Value=[-973556231.813425]  SampleTime=1
  cfblk2 : Outport
  cfblk15 : Outport  Port=2
  wires:
  cfblk9/1 -> cfblk8/1
  cfblk5/1 -> cfblk11/1(cfblk1)
  cfblk4/1 -> cfblk12/1(cfblk1)
  cfblk10/1(cfblk2) -> cfblk4/1
  cfblk1/1 -> cfblk5/1
  cfblk11/1(cfblk2) -> cfblk15/1
  cfblk14/1 -> cfblk6/1
  cfblk8/1 -> cfblk3/1
  cfblk7/1 -> cfblk13/1(cfblk1)
  cfblk3/1 -> cfblk10/1(cfblk1)
  cfblk6/1 -> cfblk2/1
  cfblk12/1(cfblk2) -> cfblk16/1
  cfblk16/1 -> cfblk3/2
  cfblk13/1(cfblk2) -> cfblk17/1
  cfblk17/1 -> cfblk7/1

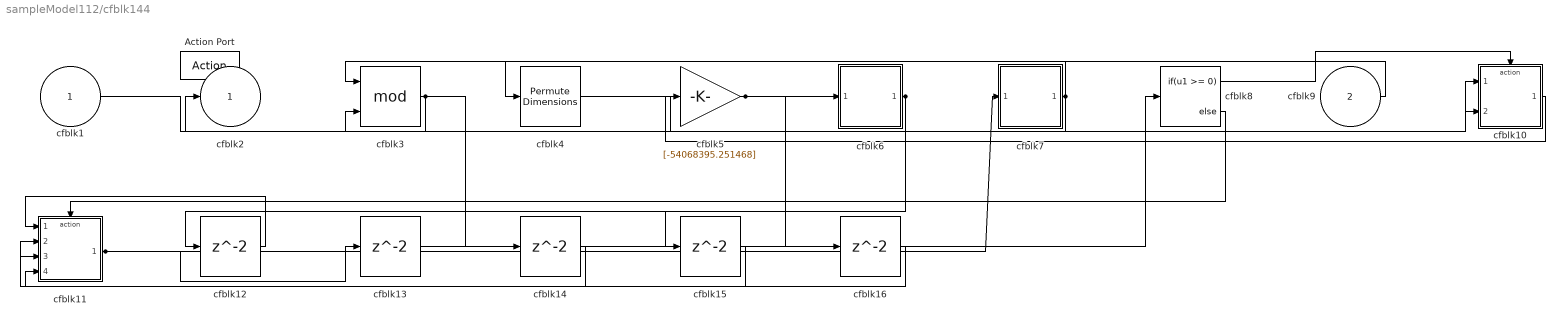
== system sampleModel112/cfblk144 ==
  cfblk1 : Inport
  cfblk9 : Inport  Port=2
  Action Port : ActionPort  ActionType=then
  cfblk10 : Subsystem  TreatAsAtomicUnit=on
  cfblk11 : Subsystem  TreatAsAtomicUnit=on
  cfblk{12..16} (5 alike) : Delay
  cfblk3 : Math  Operator=mod  SaturateOnIntegerOverflow=on
  cfblk4 : PermuteDimensions
  cfblk5 : Gain  Gain=[-54068395.251468]
  cfblk6 : Subsystem
  cfblk7 : Subsystem
  cfblk8 : If  IfExpression=u1 >= 0  SampleTime=1
  cfblk2 : Outport
  wires:
  cfblk9/1 -> cfblk4/1
  cfblk4/1 -> cfblk10/1(cfblk1)
  cfblk3/1 -> cfblk2/1, cfblk14/1
  cfblk10/1(cfblk2) -> cfblk5/1
  cfblk7/1(cfblk2) -> cfblk3/1, cfblk3/2
  cfblk1/1 -> cfblk10/2(cfblk9)
  cfblk11/1(cfblk2) -> cfblk7/1(cfblk1), cfblk13/1
  cfblk5/1 -> cfblk6/1(cfblk1), cfblk16/1
  cfblk6/1(cfblk2) -> cfblk12/1, cfblk15/1
  cfblk8/1 -> cfblk10/Action
  cfblk8/2 -> cfblk11/Action
  cfblk12/1 -> cfblk11/1(cfblk1)
  cfblk13/1 -> cfblk8/1
  cfblk14/1 -> cfblk11/4(cfblk17)
  cfblk15/1 -> cfblk11/2(cfblk15)
  cfblk16/1 -> cfblk11/3(cfblk16)

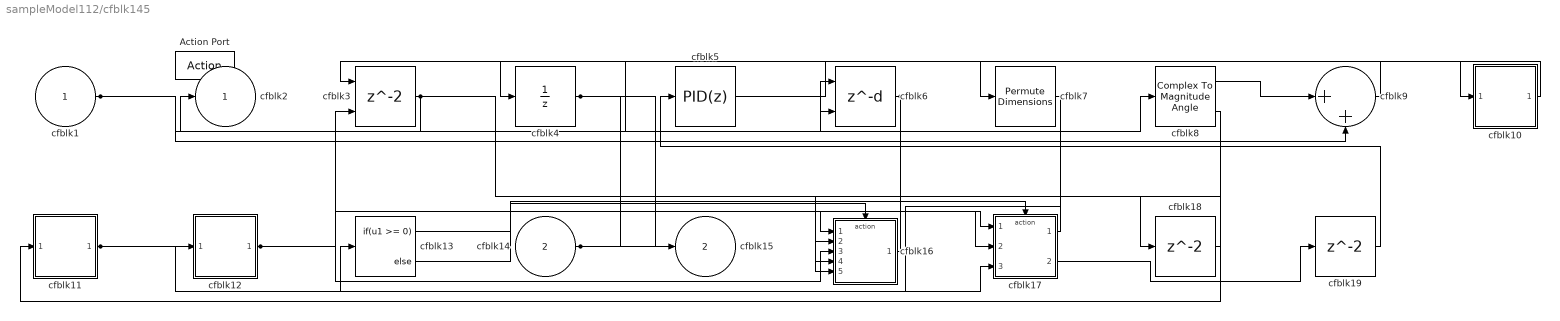
== system sampleModel112/cfblk145 ==
  cfblk1 : Inport
  cfblk14 : Inport  Port=2
  Action Port : ActionPort  ActionType=else
  cfblk10 : Subsystem
  cfblk11 : Subsystem
  cfblk12 : Subsystem
  cfblk13 : If  IfExpression=u1 >= 0  SampleTime=1
  cfblk16 : Subsystem  TreatAsAtomicUnit=on
  cfblk17 : Subsystem  TreatAsAtomicUnit=on
  cfblk18 : Delay
  cfblk19 : Delay
  cfblk3 : Delay  ShowEnablePort=on
      settings: InputPortMap=u0,e6
  cfblk4 : UnitDelay  SampleTime=-1
  cfblk5 : simulink/Continuous/PID Controller  Controller=PID  TimeDomain=Discrete-time  SampleTime=-1  IntegratorMethod=Forward Euler  FilterMethod=Forward Euler  Form=Parallel  UseFilter=on  ControllerParametersSource=internal  P=1  I=1  D=0  N=100  InitialConditionSource=internal  InitialConditionForIntegrator=0  InitialConditionForFilter=0  ExternalReset=none  LimitOutput=off  UpperSaturationLimit=inf  LowerSaturationLimit=-inf  LinearizeAsGain=off  AntiWindupMode=none  Kb=1  TrackingMode=off  Kt=1  PParamMin=[]  PParamMax=[]  IParamMin=[]  IParamMax=[]  DParamMin=[]  DParamMax=[]  NParamMin=[]  NParamMax=[]  KbParamMin=[]  KbParamMax=[]  KtParamMin=[]  KtParamMax=[]  POutMin=[]  POutMax=[]  IOutMin=[]  IOutMax=[]  DOutMin=[]  DOutMax=[]  NOutMin=[]  NOutMax=[]  KbOutMin=[]  KbOutMax=[]  KtOutMin=[]  KtOutMax=[]  IntegratorOutMin=[]  IntegratorOutMax=[]  FilterOutMin=[]  FilterOutMax=[]  SumOutMin=[]  SumOutMax=[]  SumI1OutMin=[]  SumI1OutMax=[]  SumI2OutMin=[]  SumI2OutMax=[]  SumI3OutMin=[]  SumI3OutMax=[]  SumDOutMin=[]  SumDOutMax=[]  SaturationOutMin=[]  SaturationOutMax=[]  IntegratorContinuousStateAttributes=''  IntegratorStateMustResolveToSignalObject=off  IntegratorRTWStateStorageClass=Auto  FilterContinuousStateAttributes=''  FilterStateMustResolveToSignalObject=off  FilterRTWStateStorageClass=Auto  DifferentiatorICPrevScaledInput=0  DifferentiatorOutMin=[]  DifferentiatorOutMax=[]  FilterDiffOutCoefMin=[]  FilterDiffOutCoefMax=[]  SumDenOutMin=[]  SumDenOutMax=[]  SumNumOutMin=[]  SumNumOutMax=[]  ReciprocalOutMin=[]  ReciprocalOutMax=[]  DivideOutMin=[]  DivideOutMax=[]  TunerSelectOption=Transfer Function Based (PID Tuner App)
  cfblk6 : Delay  DelayLengthSource=Input port
      settings: InputPortMap=u0,p1
  cfblk7 : PermuteDimensions
  cfblk8 : ComplexToMagnitudeAngle
  cfblk9 : Sum  Inputs=|++
  cfblk2 : Outport
  cfblk15 : Outport  Port=2
  wires:
  cfblk4/1 -> cfblk15/1, cfblk16/5(cfblk15)
  cfblk16/1(cfblk2) -> cfblk3/1
  cfblk5/1 -> cfblk10/1(cfblk1)
  cfblk3/1 -> cfblk2/1, cfblk18/1
  cfblk7/1 -> cfblk13/1
  cfblk12/1(cfblk2) -> cfblk3/2, cfblk16/3(cfblk13), cfblk17/2(cfblk7)
  cfblk11/1(cfblk2) -> cfblk12/1(cfblk1), cfblk17/3(cfblk8)
  cfblk10/1(cfblk2) -> cfblk7/1
  cfblk14/1 -> cfblk8/1, cfblk17/1(cfblk1)
  cfblk17/1(cfblk2) -> cfblk6/1
  cfblk8/1 -> cfblk9/1
  cfblk8/2 -> cfblk11/1(cfblk1)
  cfblk1/1 -> cfblk6/2, cfblk9/2
  cfblk6/1 -> cfblk16/1(cfblk1), cfblk16/4(cfblk14)
  cfblk9/1 -> cfblk4/1
  cfblk13/1 -> cfblk16/Action
  cfblk13/2 -> cfblk17/Action
  cfblk18/1 -> cfblk16/2(cfblk12)
  cfblk17/2(cfblk9) -> cfblk19/1
  cfblk19/1 -> cfblk5/1

== system sampleModel112/cfblk146 ==
  cfblk1 : Inport
  Action Port : ActionPort  ActionType=then
  cfblk3 : Sum  Inputs=+-
  cfblk4 : ComplexToMagnitudeAngle
  cfblk5 : Subsystem
  cfblk6 : Subsystem
  cfblk8 : Delay
  cfblk2 : Outport
  cfblk7 : Outport  Port=2
  wires:
  cfblk5/1(cfblk2) -> cfblk3/1
  cfblk3/1 -> cfblk4/1
  cfblk4/1 -> cfblk7/1
  cfblk4/2 -> cfblk6/1(cfblk1)
  cfblk1/1 -> cfblk5/1(cfblk1)
  cfblk6/1(cfblk2) -> cfblk2/1, cfblk8/1
  cfblk8/1 -> cfblk3/2

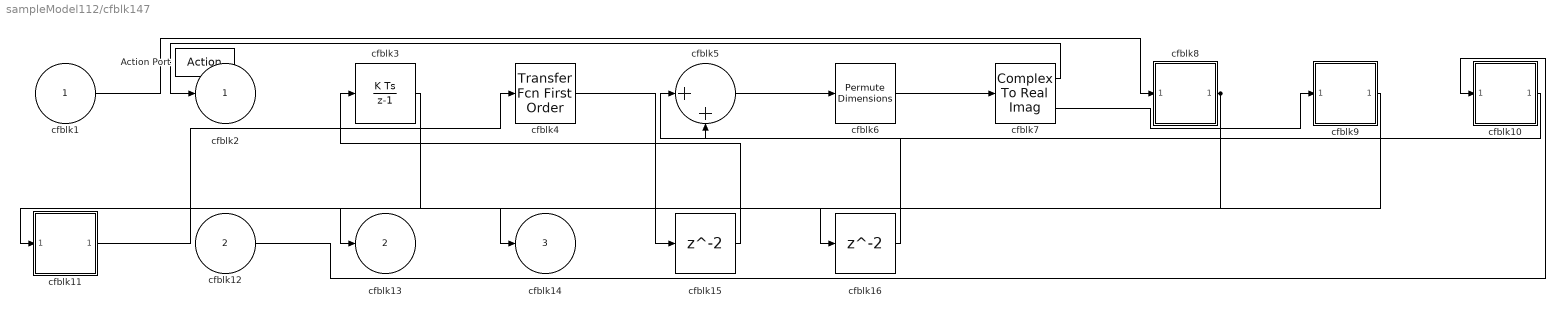
== system sampleModel112/cfblk147 ==
  cfblk1 : Inport
  cfblk12 : Inport  Port=2
  Action Port : ActionPort  ActionType=else
  cfblk10 : Subsystem
  cfblk11 : Subsystem
  cfblk15 : Delay
  cfblk16 : Delay
  cfblk3 : DiscreteIntegrator  SampleTime=-1  ICPrevOutput=DiscIntNeverNeededParam  ICPrevScaledInput=DiscIntNeverNeededParam
  cfblk4 : simulink/Discrete/Transfer Fcn First Order  PoleZ=0.95  ICPrevOutput=0.0  DoSatur=off
      settings: SourceProductName=Simulink
  cfblk5 : Sum  Inputs=|++
  cfblk6 : PermuteDimensions
  cfblk7 : ComplexToRealImag
  cfblk8 : Subsystem
  cfblk9 : Subsystem
  cfblk2 : Outport
  cfblk13 : Outport  Port=2
  cfblk14 : Outport  Port=3
  wires:
  cfblk3/1 -> cfblk11/1(cfblk1)
  cfblk7/1 -> cfblk2/1
  cfblk1/1 -> cfblk8/1(cfblk1)
  cfblk7/2 -> cfblk9/1(cfblk1)
  cfblk6/1 -> cfblk7/1
  cfblk10/1(cfblk2) -> cfblk5/1
  cfblk8/1(cfblk2) -> cfblk13/1, cfblk14/1
  cfblk11/1(cfblk2) -> cfblk4/1
  cfblk12/1 -> cfblk10/1(cfblk1)
  cfblk5/1 -> cfblk6/1
  cfblk4/1 -> cfblk15/1
  cfblk15/1 -> cfblk3/1
  cfblk9/1(cfblk2) -> cfblk16/1
  cfblk16/1 -> cfblk5/2

== system sampleModel112/cfblk130/cfblk5 ==
  cfblk1 : Inport
  cfblk2 : Outport
  wires:
  cfblk1/1 -> cfblk2/1

== system sampleModel112/cfblk131/cfblk11 ==
  cfblk1 : Inport
  Action Port : ActionPort  ActionType=then
  cfblk3 : DiscreteIntegrator  SampleTime=-1  ICPrevOutput=DiscIntNeverNeededParam  ICPrevScaledInput=DiscIntNeverNeededParam
  cfblk4 : DiscreteStateSpace  SampleTime=-1
  cfblk5 : ComplexToMagnitudeAngle
  cfblk6 : Product  Inputs=**
  cfblk7 : Subsystem
  cfblk8 : Delay
  cfblk2 : Outport
  wires:
  cfblk7/1(cfblk2) -> cfblk6/1
  cfblk4/1 -> cfblk7/1(cfblk1)
  cfblk5/2 -> cfblk3/1
  cfblk6/1 -> cfblk5/1
  cfblk1/1 -> cfblk4/1
  cfblk3/1 -> cfblk2/1
  cfblk5/1 -> cfblk8/1
  cfblk8/1 -> cfblk6/2

== system sampleModel112/cfblk131/cfblk12 ==
  cfblk1 : Inport
  cfblk8 : Inport  Port=2
  Action Port : ActionPort  ActionType=else
  cfblk3 : UnitDelay  SampleTime=-1
  cfblk4 : DiscreteZeroPole  Poles=[0 0.5]  Gain=1  SampleTime=-1
  cfblk5 : DiscreteZeroPole  Poles=[0 0.5]  Gain=1  SampleTime=-1
  cfblk6 : Product
  cfblk7 : Sum  Inputs=+-
  cfblk2 : Outport
  wires:
  cfblk3/1 -> cfblk6/1
  cfblk8/1 -> cfblk3/1, cfblk5/1
  cfblk4/1 -> cfblk6/2
  cfblk7/1 -> cfblk4/1
  cfblk1/1 -> cfblk7/1
  cfblk5/1 -> cfblk7/2
  cfblk6/1 -> cfblk2/1

== system sampleModel112/cfblk131/cfblk7 ==
  cfblk1 : Inport
  cfblk2 : Outport
  wires:
  cfblk1/1 -> cfblk2/1

== system sampleModel112/cfblk131/cfblk8 ==
  cfblk1 : Inport
  cfblk2 : Outport
  wires:
  cfblk1/1 -> cfblk2/1

== system sampleModel112/cfblk132/cfblk10 ==
  cfblk1 : Inport
  cfblk2 : Outport
  wires:
  cfblk1/1 -> cfblk2/1

== system sampleModel112/cfblk132/cfblk11 ==
  cfblk1 : Inport
  cfblk2 : Outport
  wires:
  cfblk1/1 -> cfblk2/1

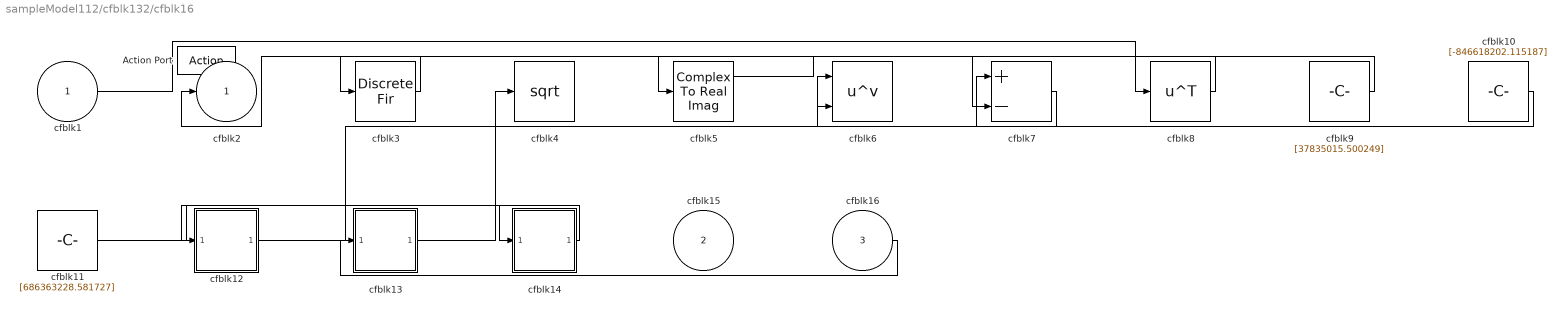
== system sampleModel112/cfblk132/cfblk16 ==
  cfblk1 : Inport
  cfblk15 : Inport  Port=2
  cfblk16 : Inport  Port=3
  Action Port : ActionPort  ActionType=then
  cfblk10 : Constant  Value=[-846618202.115187]  SampleTime=1
  cfblk11 : Constant  Value=[686363228.581727]  SampleTime=1
  cfblk12 : Subsystem
  cfblk13 : Subsystem
  cfblk14 : Subsystem
  cfblk3 : DiscreteFir
  cfblk4 : Sqrt  SaturateOnIntegerOverflow=on
  cfblk5 : ComplexToRealImag
  cfblk6 : Math  Operator=pow  SaturateOnIntegerOverflow=on
  cfblk7 : Sum  Inputs=+-
  cfblk8 : Math  Operator=transpose  SaturateOnIntegerOverflow=on
  cfblk9 : Constant  Value=[37835015.500249]  SampleTime=1
  cfblk2 : Outport
  wires:
  cfblk12/1(cfblk2) -> cfblk6/1
  cfblk1/1 -> cfblk8/1
  cfblk3/1 -> cfblk2/1
  cfblk10/1 -> cfblk7/1
  cfblk16/1 -> cfblk13/1(cfblk1)
  cfblk11/1 -> cfblk14/1(cfblk1)
  cfblk13/1(cfblk2) -> cfblk4/1
  cfblk8/1 -> cfblk3/1
  cfblk14/1(cfblk2) -> cfblk12/1(cfblk1)
  cfblk7/1 -> cfblk6/2
  cfblk9/1 -> cfblk5/1
  cfblk5/1 -> cfblk7/2

== system sampleModel112/cfblk132/cfblk17 ==
  cfblk1 : Inport
  cfblk8 : Inport  Port=2
  Action Port : ActionPort  ActionType=else
  cfblk3 : DiscreteStateSpace  SampleTime=-1
  cfblk4 : Rounding
  cfblk5 : Subsystem
  cfblk6 : Subsystem
  cfblk7 : Subsystem
  cfblk2 : Outport
  cfblk9 : Outport  Port=2
  wires:
  cfblk8/1 -> cfblk5/1(cfblk1)
  cfblk5/1(cfblk2) -> cfblk6/1(cfblk1)
  cfblk1/1 -> cfblk2/1
  cfblk4/1 -> cfblk9/1
  cfblk3/1 -> cfblk4/1
  cfblk7/1(cfblk2) -> cfblk3/1
  cfblk6/1(cfblk2) -> cfblk7/1(cfblk1)
